simulink model "pmsm_model_1"  (R2023a)
settings: Solver=VariableStepAuto  StartTime=0.0  StopTime=10.0  RelTol=1e-3
settings Model: Creator=Atharva  LastModifiedBy=Atharva

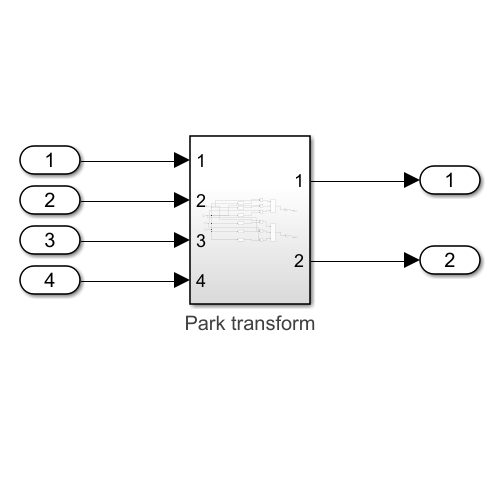
[thumbnail: Simulink's stored preview of the top-level diagram]
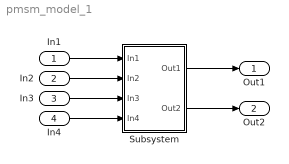
== system pmsm_model_1 ==
  In1 : Inport  Tag=Va
  In2 : Inport  Port=2
  In3 : Inport  Port=3
  In4 : Inport  Port=4
  Subsystem : Subsystem
      settings: AttributesFormatString=Park transform
  Out1 : Outport
  Out2 : Outport  Port=2
  wires:
  In1/1 -> Subsystem/1(In1)
  In2/1 -> Subsystem/2(In2)
  In3/1 -> Subsystem/3(In3)
  In4/1 -> Subsystem/4(In4)
  Subsystem/1(Out1) -> Out1/1
  Subsystem/2(Out2) -> Out2/1

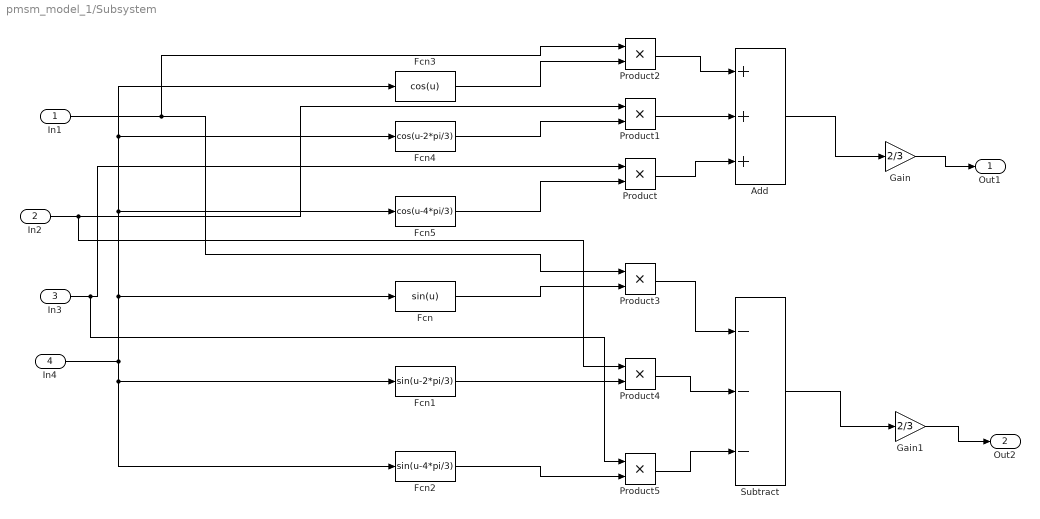
== system pmsm_model_1/Subsystem ==
  In1 : Inport  Tag=Va
  In2 : Inport  Port=2
  In3 : Inport  Port=3
  In4 : Inport  Port=4
  Add : Sum  Inputs=+++
  Fcn : Fcn  Expr=sin(u)
  Fcn1 : Fcn  Expr=sin(u-2*pi/3)
  Fcn2 : Fcn  Expr=sin(u-4*pi/3)
  Fcn3 : Fcn  Expr=cos(u)
  Fcn4 : Fcn  Expr=cos(u-2*pi/3)
  Fcn5 : Fcn  Expr=cos(u-4*pi/3)
  Gain : Gain  Gain=2/3
  Gain1 : Gain  Gain=2/3
  Product{,1..5} (6 alike) : Product
  Subtract : Sum  Inputs=---
  Out1 : Outport
  Out2 : Outport  Port=2
  wires:
  Product3/1 -> Subtract/1
  Product2/1 -> Add/1
  In3/1 -> Product5/1, Product/1
  Product/1 -> Add/3
  Add/1 -> Gain/1
  Fcn1/1 -> Product4/2
  In4/1 -> Fcn/1, Fcn4/1, Fcn3/1, Fcn5/1, Fcn2/1, Fcn1/1
  Fcn3/1 -> Product2/2
  Gain/1 -> Out1/1
  Subtract/1 -> Gain1/1
  Product1/1 -> Add/2
  Fcn4/1 -> Product1/2
  Product4/1 -> Subtract/2
  Product5/1 -> Subtract/3
  Fcn/1 -> Product3/2
  In1/1 -> Product2/1, Product3/1
  Gain1/1 -> Out2/1
  Fcn5/1 -> Product/2
  In2/1 -> Product4/1, Product1/1
  Fcn2/1 -> Product5/2
